simulink model "Blsaturetion"  (R2021a)
settings: Solver=FixedStepDiscrete  StartTime=0.0  StopTime=10.0  FixedStep=0.1  RelTol=1e-3
settings Model: Creator=mymind  LastModifiedBy=mymind

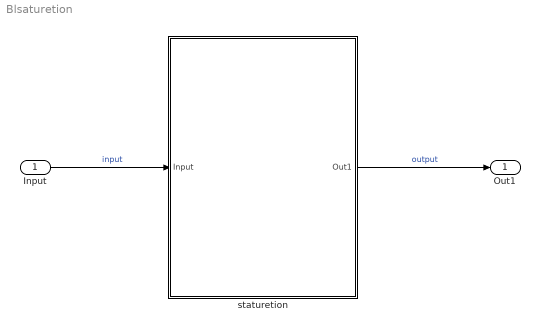
== system Blsaturetion ==
  Input : Inport
  staturetion : Subsystem
  Out1 : Outport
  wires:
  Input/1 -> staturetion/1(Input)  "input"
  staturetion/1(Out1) -> Out1/1  "output"

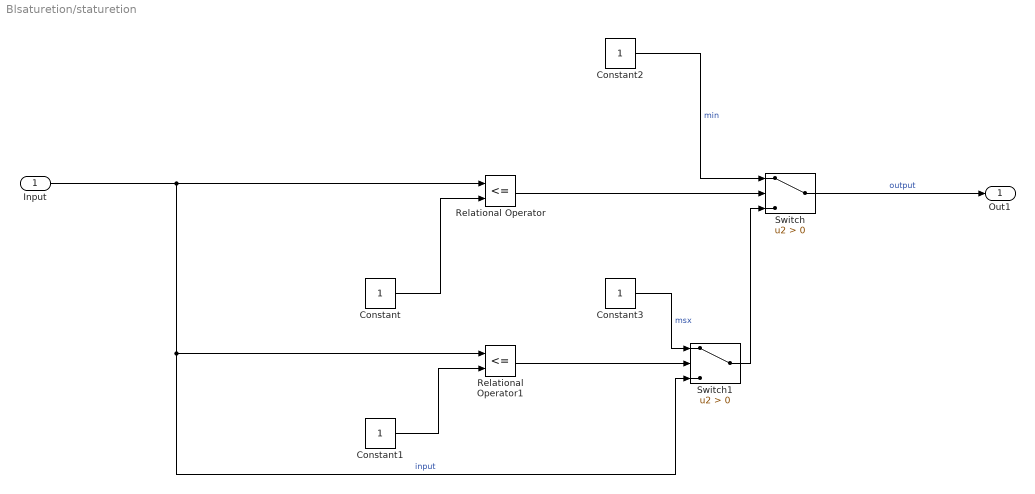
== system Blsaturetion/staturetion ==
  Input : Inport
  Constant{,1..3} (4 alike) : Constant
  Relational Operator : RelationalOperator  Operator=<=  OutDataTypeStr=boolean  RndMeth=Simplest
  Relational Operator1 : RelationalOperator  Operator=<=  OutDataTypeStr=boolean  RndMeth=Simplest
  Switch : Switch  Criteria=u2 > Threshold
  Switch1 : Switch  Criteria=u2 > Threshold
  Out1 : Outport
  wires:
  Switch/1 -> Out1/1  "output"
  Switch1/1 -> Switch/3
  Relational Operator/1 -> Switch/2
  Relational Operator1/1 -> Switch1/2
  Constant1/1 -> Relational Operator1/2
  Constant/1 -> Relational Operator/2
  Constant2/1 -> Switch/1  "min"
  Constant3/1 -> Switch1/1  "msx"
  Input/1 -> Switch1/3, Relational Operator1/1, Relational Operator/1  "input"
